simulink model "mpcModel"  (R2020a)
settings: Solver=VariableStepAuto  StartTime=0.0  StopTime=10.0  FixedStep=Ts  RelTol=1e-3
undefined symbols (not defined in the file): A, B, C, ref, sysm, Ts
libraries: mympclib x2
settings Model: Creator=kohei  LastModifiedBy=kohei
settings DataIOCC: ReturnWorkspaceOutputs=off
settings OptimizationCC: DefaultParameterBehavior=Inlined  EnhancedBackFolding=on  PassReuseOutputArgsAs=Individual arguments  ZeroExternalMemoryAtStartup=off  ZeroInternalMemoryAtStartup=off  OptimizeBlockOrder=speed  DifferentSizesBufferReuse=on  OptimizationCustomize=off  EfficientTunableParamExpr=on
settings DebuggingCC: ParameterTunabilityLossMsg=error
settings SFSimCC: MATLABDynamicMemAlloc=off
settings RTWCC: SystemTargetFile=ert.tlc  TemplateMakefile=ert_default_tmf
settings CodeAppCC: ForceParamTrailComments=on  IgnoreCustomStorageClasses=off  OperatorAnnotations=on  SimulinkDataObjDesc=on  SFDataObjDesc=on  InsertBlockDesc=on
settings ERTTargetCC: TargetLangStandard=C99 (ISO)  GenerateSampleERTMain=on  SupportVariableSizeSignals=on  InlinedParameterPlacement=NonHierarchical  ERTCustomFileTemplate=example_file_process.tlc

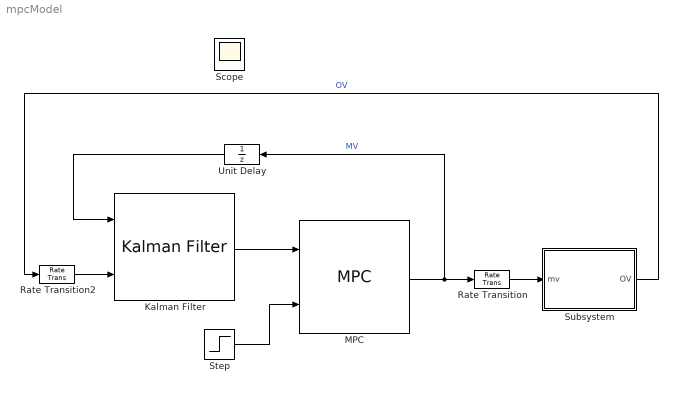
== system mpcModel ==
  Kalman Filter : mympclib/Kalman Filter  A=sysm.A  Bu=sysm.B  Bv=1  C=sysm.C  Q=1  R=0.1  xhat0=0  P0=1  Ts=Ts  enableP=off  enableG=off
      settings: SourceProductName=My MPC Library
  MPC : mympclib/MPC  params=params  sysm=sysm  numState=1  numRef=1  numMV=1  Ts=Ts  enableDist=off  numDist=1  enableSlack=off  enableStatus=off  enableMVseq=off
      settings: SourceProductName=My MPC Library
  Rate Transition : RateTransition
  Rate Transition2 : RateTransition
  Step : Step  After=ref  SampleTime=Ts
  Subsystem : Subsystem
  Unit Delay : UnitDelay  SampleTime=-1  HasFrameUpgradeWarning=on
  Scope : Scope
  wires:
  MPC/1 -> Rate Transition/1, Unit Delay/1  "MV"
  Subsystem/1(OV) -> Rate Transition2/1  "OV"
  Rate Transition/1 -> Subsystem/1(mv)
  Rate Transition2/1 -> Kalman Filter/2
  Unit Delay/1 -> Kalman Filter/1
  Kalman Filter/1 -> MPC/1
  Step/1 -> MPC/2

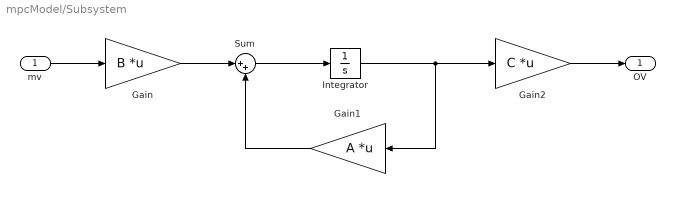
== system mpcModel/Subsystem ==
  mv : Inport
  Gain : Gain  Gain=B  Multiplication=Matrix(K*u) (u vector)
  Gain1 : Gain  Gain=A  Multiplication=Matrix(K*u) (u vector)
  Gain2 : Gain  Gain=C  Multiplication=Matrix(K*u) (u vector)
  Integrator : Integrator
  Sum : Sum  Inputs=|++
  OV : Outport
  wires:
  Gain1/1 -> Sum/2
  Gain/1 -> Sum/1
  Gain2/1 -> OV/1
  Integrator/1 -> Gain1/1, Gain2/1
  Sum/1 -> Integrator/1
  mv/1 -> Gain/1
